simulink model "lab6"  (R2015a)
settings: Solver=ode45  StartTime=0.0  StopTime=630  RelTol=1e-3
undefined symbols (not defined in the file or in its folder): currentCFG_lab6_UB, UB
libraries: gtecHighspeedLib x1, gUSBamplib x1
settings Model: Creator=circuit  LastModifiedBy=circuit

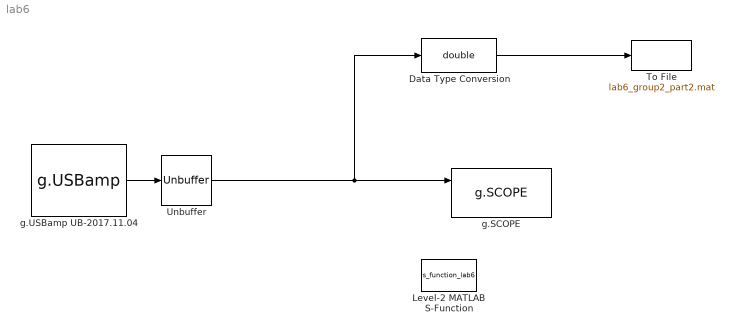
== system lab6 ==
  Data Type Conversion : DataTypeConversion  OutDataTypeStr=double
  Level-2 MATLAB S-Function : M-S-Function  FunctionName=s_function_lab6
  To File : ToFile  Filename=lab6_group2_part2.mat
  Unbuffer : Unbuffer  SampleBasedProcessing=Same as frame based
  g.SCOPE : gtecHighspeedLib/g.SCOPE
  g.USBamp UB-2017.11.04 : gUSBamplib/g.USBamp  cfg=currentCFG_lab6_UB-2017.11.04.cfg  snr=UB-2017.11.04
  wires:
  g.USBamp UB-2017.11.04/1 -> Unbuffer/1
  Data Type Conversion/1 -> To File/1
  Unbuffer/1 -> Data Type Conversion/1, g.SCOPE/1
